simulink model "single_phase_inverter_with_inductive_load_Unipolar"  (R2020a)
settings: Solver=VariableStepAuto  StartTime=0.0  StopTime=.06  MaxStep=1e-5  RelTol=1e-3
libraries: powerlib x11, powerlib_meascontrol x3, simulink x2
settings Model: Creator=User  LastModifiedBy=User

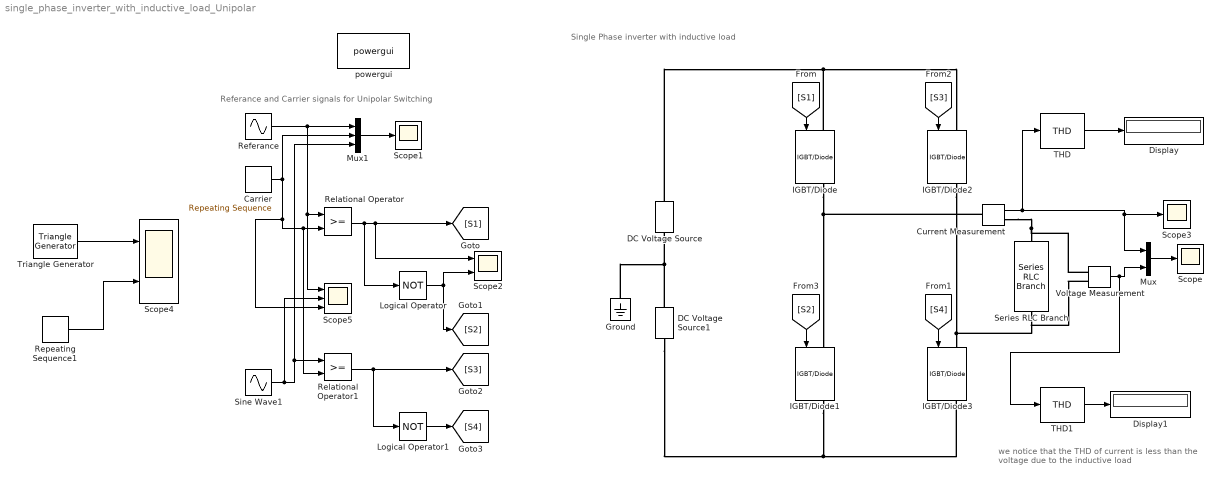
== system single_phase_inverter_with_inductive_load_Unipolar ==
  note: Referance and Carrier signals for Unipolar Switching
  note: we notice that the THD of current is less than the voltage due to the inductive load
  note: Single Phase inverter with inductive load
  Carrier : simulink/Sources/Repeating Sequence  rep_seq_t=[0 1 2 3 4]*[1/5000]  rep_seq_y=[0 1 0 -1 0]
  Current Measurement : powerlib/Measurements/Current Measurement  PhasorSimulation=off  OutputType=Complex  PSBequivalent=0
  DC Voltage Source : powerlib/Electrical Sources/DC Voltage Source  Amplitude=100  Measurements=None
  DC Voltage Source1 : powerlib/Electrical Sources/DC Voltage Source  Amplitude=100  Measurements=None
  Display : Display
  Display1 : Display
  Ground : powerlib/Elements/Ground  LConnTagsString=a
  IGBT/Diode{,1..3} (4 alike) : powerlib/Power Electronics/IGBT//Diode  Ron=1e-3  Rs=1e5  Cs=inf  Measurements=on
  Logical Operator : Logic  Operator=NOT  AllPortsSameDT=off  OutDataTypeStr=boolean
  Logical Operator1 : Logic  Operator=NOT  AllPortsSameDT=off  OutDataTypeStr=boolean
  Mux : Mux  Inputs=2
  Mux1 : Mux  Inputs=3
  Referance : Sin  Frequency=2*pi*50  SampleTime=0
  Relational Operator : RelationalOperator  OutDataTypeStr=boolean  RndMeth=Simplest
  Relational Operator1 : RelationalOperator  OutDataTypeStr=boolean  RndMeth=Simplest
  "Repeating Sequence1  " : simulink/Sources/Repeating Sequence  rep_seq_t=[0 1 2 3 4]*[1/400]  rep_seq_y=[0 1 0 -1 0]
  Scope : Scope
  Scope1 : Scope
  Scope2 : Scope  NumInputPorts=2
  Scope3 : Scope
  Scope4 : Scope  NumInputPorts=2
  Scope5 : Scope  NumInputPorts=3
  Series RLC Branch : powerlib/Elements/Series RLC Branch  LConnTagsString=__new0  RConnTagsString=__new0  BranchType=RL  Resistance=1  Inductance=50e-3  SetiL0=off  InitialCurrent=0  Capacitance=1e-6  Setx0=off  InitialVoltage=0  Measurements=None
  Sine Wave1 : Sin  Frequency=2*pi*50  Phase=pi  SampleTime=0
  THD : powerlib_meascontrol/Measurements/THD  Freq=60  Ts=0
  THD1 : powerlib_meascontrol/Measurements/THD  Freq=60  Ts=0
  "Triangle Generator " : powerlib_meascontrol/Pulse & Signal Generators/Triangle Generator  Freq=1e2  Phase=0  Ts=0
  Voltage Measurement : powerlib/Measurements/Voltage Measurement  PhasorSimulation=off  OutputType=Complex  PSBequivalent=0
  powergui : powerlib/powergui  Priority=1  SimulationMode=Continuous  SampleTime=50e-6  frequency=60  Iterations=50  frequencyindice=0  Pbase=100e6  ErrMax=1e-4  UnitsV=kV  UnitsW=MW  buscounter=0  FunctionMessages=off  echomessages=off  EnableUseOfTLC=off  CurrentSourceSwitches=off  DisableSnubberDevices=on  DisableRonSwitches=on  DisableVfSwitches=on  DisplayEquations=off  AutomaticDiscreteSolvers=off  SolverType=Tustin/Backward Euler (TBE)  Interpol=off  ExternalGateDelay=off  methode=off  Ts=100  x0status=blocks  SPID=on  SwTol=0  HookPort=off  NonlinearTolerance=1e-4  nMaxIteration=100  ContinueOnMaxIteration=off  RestoreLinks=warning  ResistiveCurrentMeasurement=off  Frange=[0:2:500]  Ylog=off  Xlog=on  ShowGrid=off  save=off  variable=ZData  structure=0  ZoomFFT=off  StartTime=0.0  cycles=1  DisplayStyle=1  fundamental=60  FreqAxis=off  MaxFrequency=1000  frequencyindicesteady=1  RmsSteady=1  display=off
  wires:
  [S1] -> IGBT/Diode/1
  [S4] -> IGBT/Diode3/1
  [S3] -> IGBT/Diode2/1
  [S2] -> IGBT/Diode1/1
  Current Measurement/1 -> Mux/1, Scope3/1, THD/1
  Voltage Measurement/1 -> THD1/1, Mux/2
  Mux/1 -> Scope/1
  THD/1 -> Display/1
  THD1/1 -> Display1/1
  Referance/1 -> Scope5/1, Relational Operator/1, Mux1/1
  Carrier/1 -> Scope5/3, Relational Operator1/2, Relational Operator/2, Mux1/2
  Mux1/1 -> Scope1/1
  Relational Operator/1 -> [S1], Scope2/1, Logical Operator/1
  Logical Operator/1 -> [S2], Scope2/2
  Relational Operator1/1 -> Logical Operator1/1, [S3]
  Logical Operator1/1 -> [S4]
  "Triangle Generator "/1 -> Scope4/1
  "Repeating Sequence1  "/1 -> Scope4/2
  Sine Wave1/1 -> Scope5/2, Mux1/3, Relational Operator1/1
  connections:
  IGBT/Diode/LConn1 -- DC Voltage Source/RConn1 -- IGBT/Diode2/LConn1
  IGBT/Diode1/RConn1 -- DC Voltage Source1/LConn1 -- IGBT/Diode3/RConn1
  IGBT/Diode2/RConn1 -- Voltage Measurement/LConn2 -- Series RLC Branch/RConn1 -- IGBT/Diode3/LConn1
  IGBT/Diode/RConn1 -- Current Measurement/LConn1 -- IGBT/Diode1/LConn1
  DC Voltage Source1/RConn1 -- Ground/LConn1 -- DC Voltage Source/LConn1
  Current Measurement/RConn1 -- Voltage Measurement/LConn1 -- Series RLC Branch/LConn1
